simulink model "WelcomeFwdStEnCtrl"  (R2018b)
settings: Solver=FixedStepDiscrete  StartTime=0.0  StopTime=10.0  FixedStep=0.01  RelTol=1e-3
undefined symbols (not defined in the file or in its folder): data, KeSMSw4SSecRwLtStLgrstOtwdInwdClosePos1_Val, KeSMSw4SSecRwLtStLgrstUpwdDnwdClosePos1_Val, KeSMSw4SSecRwLtStLgrstUpwdDnwdClosePos2_Val, KeSMSw4SSecRwRtStLgrstOtwdInwdClosePos1_Val, KeSMSw4SSecRwRtStLgrstUpwdDnwdClosePos1_Val, KeSMSw4SSecRwRtStLgrstUpwdDnwdClosePos2_Val, SecRwLtStBkReclnEn_Clear, SecRwLtStBkReclnEn_Set, SecRwLtStFtrstEn_Clear, SecRwLtStFtrstEn_Set, SecRwLtStFwdBkwdEn_Clear, SecRwLtStFwdBkwdEn_Set, SecRwLtStHdrstFwdBkwdEn_Clear, SecRwLtStHdrstFwdBkwdEn_Set, SecRwLtStHdrstUpwdDnwdEn_Clear, SecRwLtStHdrstUpwdDnwdEn_Set, SecRwLtStLgrstInwdOtwdEn_Clear, SecRwLtStLgrstInwdOtwdEn_Set, SecRwLtStLgrstUpwdDnwdEn_Clear, SecRwLtStLgrstUpwdDnwdEn_Set, SecRwRtStBkReclnEn_Clear, SecRwRtStBkReclnEn_Set, SecRwRtStFtrstEn_Clear, SecRwRtStFtrstEn_Set, SecRwRtStFwdBkwdEn_Clear, SecRwRtStFwdBkwdEn_Set, SecRwRtStHdrstFwdBkwdEn_Clear, SecRwRtStHdrstFwdBkwdEn_Set, SecRwRtStHdrstUpwdDnwdEn_Clear, SecRwRtStHdrstUpwdDnwdEn_Set, SecRwRtStLgrstInwdOtwdEn_Clear, SecRwRtStLgrstInwdOtwdEn_Set, SecRwRtStLgrstUpwdDnwdEn_Clear, SecRwRtStLgrstUpwdDnwdEn_Set
libraries: simulink x1
settings Model: ModifiedHistory=2023.8.1 V2.0.0 CR421790 增加模式21-26  Creator=sn2xws  LastModifiedBy=sn2xws
settings DataIOCC: SaveFormat=StructureWithTime
settings OptimizationCC: DefaultParameterBehavior=Inlined  EnhancedBackFolding=on  PassReuseOutputArgsAs=Individual arguments  ZeroExternalMemoryAtStartup=off  ZeroInternalMemoryAtStartup=off  OptimizeBlockOrder=speed  DifferentSizesBufferReuse=on  OptimizationCustomize=off
settings DebuggingCC: ParameterTunabilityLossMsg=error
settings SFSimCC: MATLABDynamicMemAlloc=off
settings RTWCC: SystemTargetFile=autosar.tlc  GenCodeOnly=on  TemplateMakefile=ert_default_tmf  Description=AUTOSAR  GenerateReport=on  IncludeHyperlinkInReport=on  LaunchReport=on  GenerateTraceInfo=on  GenerateTraceReport=on  GenerateTraceReportSl=on  GenerateTraceReportSf=on  GenerateTraceReportEml=on  GenerateCodeMetricsReport=on
settings CodeAppCC: ForceParamTrailComments=on  IgnoreCustomStorageClasses=off  OperatorAnnotations=on  SimulinkDataObjDesc=on  SFDataObjDesc=on  InsertBlockDesc=on
settings STFCustomTargetCC: TargetLangStandard=C99 (ISO)  MultiwordLength=256  ParMdlRefBuildCompliant=on  CompOptLevelCompliant=on  IncludeMdlTerminateFcn=off  CombineOutputUpdateFcns=on  SuppressErrorStatus=on  ERTCustomFileBanners=on  SupportNonFinite=off  SupportComplex=off  SupportContinuousTime=off  SupportNonInlinedSFcns=off  RemoveResetFunc=on  MATLABClassNameForMDSCustomization=Simulink.SoftwareTarget.ERTCustomization  AutosarCompliant=on  UseToolchainInfoCompliant=on  LookupTableObjectStructAxisOrder=2,1,3,4,...  LUTObjectStructOrderEvenSpacing=Size,Table,Breakpoints  SystemTargetFile=autosar.tlc
settings ERTTargetCC: TargetLangStandard=C99 (ISO)  ConcurrentExecutionCompliant=off  IncludeMdlTerminateFcn=off  SuppressErrorStatus=on  SupportNonFinite=off  SupportComplex=off  ModelStepFunctionPrototypeControlCompliant=off  CPPClassGenCompliant=off  AutosarCompliant=on  LookupTableObjectStructAxisOrder=2,1,3,4,...  LUTObjectStructOrderEvenSpacing=Size,Table,Breakpoints  InlinedParameterPlacement=NonHierarchical  ERTCustomFileTemplate=example_file_process.tlc  ERTFilePackagingFormat=Compact

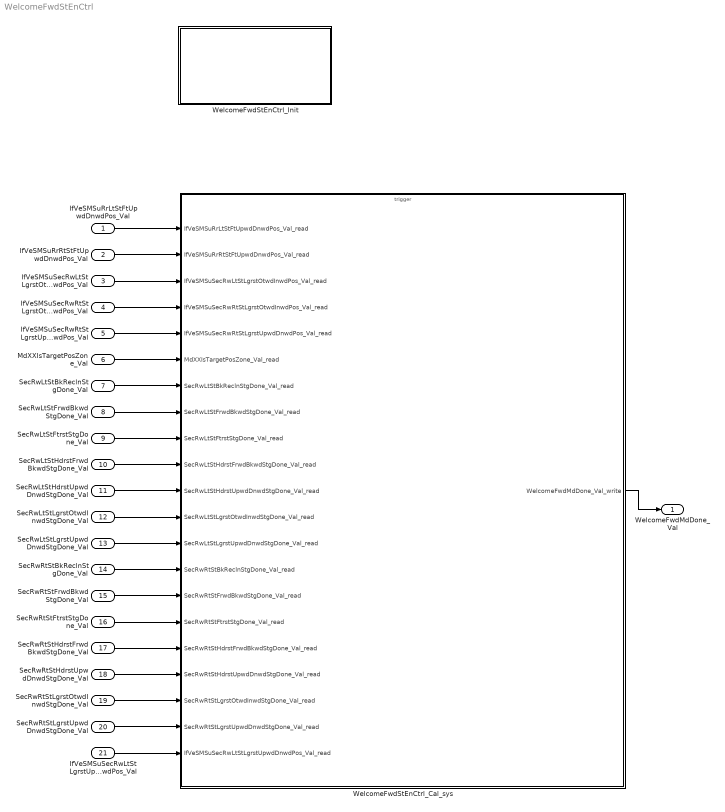
== system WelcomeFwdStEnCtrl ==
  IfVeSMSuRrLtStFtUpwdDnwdPos_Val : Inport  OutDataTypeStr=uint16  PortDimensions=1
  IfVeSMSuRrRtStFtUpwdDnwdPos_Val : Inport  Port=2  OutDataTypeStr=uint16  PortDimensions=1
  IfVeSMSuSecRwLtStLgrstOtwdInwdPos_Val : Inport  Port=3  OutDataTypeStr=uint16  PortDimensions=1
  IfVeSMSuSecRwRtStLgrstOtwdInwdPos_Val : Inport  Port=4  OutDataTypeStr=uint16  PortDimensions=1
  IfVeSMSuSecRwRtStLgrstUpwdDnwdPos_Val : Inport  Port=5  OutDataTypeStr=uint16  PortDimensions=1
  MdXXIsTargetPosZone_Val : Inport  Port=6  OutDataTypeStr=uint32  PortDimensions=1
  SecRwLtStBkReclnStgDone_Val : Inport  Port=7  OutDataTypeStr=boolean  PortDimensions=1
  SecRwLtStFrwdBkwdStgDone_Val : Inport  Port=8  OutDataTypeStr=boolean  PortDimensions=1
  SecRwLtStFtrstStgDone_Val : Inport  Port=9  OutDataTypeStr=boolean  PortDimensions=1
  SecRwLtStHdrstFrwdBkwdStgDone_Val : Inport  Port=10  OutDataTypeStr=boolean  PortDimensions=1
  SecRwLtStHdrstUpwdDnwdStgDone_Val : Inport  Port=11  OutDataTypeStr=boolean  PortDimensions=1
  SecRwLtStLgrstOtwdInwdStgDone_Val : Inport  Port=12  OutDataTypeStr=boolean  PortDimensions=1
  SecRwLtStLgrstUpwdDnwdStgDone_Val : Inport  Port=13  OutDataTypeStr=boolean  PortDimensions=1
  SecRwRtStBkReclnStgDone_Val : Inport  Port=14  OutDataTypeStr=boolean  PortDimensions=1
  SecRwRtStFrwdBkwdStgDone_Val : Inport  Port=15  OutDataTypeStr=boolean  PortDimensions=1
  SecRwRtStFtrstStgDone_Val : Inport  Port=16  OutDataTypeStr=boolean  PortDimensions=1
  SecRwRtStHdrstFrwdBkwdStgDone_Val : Inport  Port=17  OutDataTypeStr=boolean  PortDimensions=1
  SecRwRtStHdrstUpwdDnwdStgDone_Val : Inport  Port=18  OutDataTypeStr=boolean  PortDimensions=1
  SecRwRtStLgrstOtwdInwdStgDone_Val : Inport  Port=19  OutDataTypeStr=boolean  PortDimensions=1
  SecRwRtStLgrstUpwdDnwdStgDone_Val : Inport  Port=20  OutDataTypeStr=boolean  PortDimensions=1
  IfVeSMSuSecRwLtStLgrstUpwdDnwdPos_Val : Inport  Port=21  OutDataTypeStr=uint16  PortDimensions=1
  WelcomeFwdStEnCtrl_Cal_sys : Subsystem
  WelcomeFwdStEnCtrl_Init : Subsystem
  WelcomeFwdMdDone_Val : Outport  OutDataTypeStr=uint8  PortDimensions=1
  wires:
  IfVeSMSuRrLtStFtUpwdDnwdPos_Val/1 -> WelcomeFwdStEnCtrl_Cal_sys/1(IfVeSMSuRrLtStFtUpwdDnwdPos_Val_read)
  IfVeSMSuRrRtStFtUpwdDnwdPos_Val/1 -> WelcomeFwdStEnCtrl_Cal_sys/2(IfVeSMSuRrRtStFtUpwdDnwdPos_Val_read)
  IfVeSMSuSecRwLtStLgrstOtwdInwdPos_Val/1 -> WelcomeFwdStEnCtrl_Cal_sys/3(IfVeSMSuSecRwLtStLgrstOtwdInwdPos_Val_read)
  IfVeSMSuSecRwRtStLgrstOtwdInwdPos_Val/1 -> WelcomeFwdStEnCtrl_Cal_sys/4(IfVeSMSuSecRwRtStLgrstOtwdInwdPos_Val_read)
  IfVeSMSuSecRwRtStLgrstUpwdDnwdPos_Val/1 -> WelcomeFwdStEnCtrl_Cal_sys/5(IfVeSMSuSecRwRtStLgrstUpwdDnwdPos_Val_read)
  MdXXIsTargetPosZone_Val/1 -> WelcomeFwdStEnCtrl_Cal_sys/6(MdXXIsTargetPosZone_Val_read)
  SecRwLtStBkReclnStgDone_Val/1 -> WelcomeFwdStEnCtrl_Cal_sys/7(SecRwLtStBkReclnStgDone_Val_read)
  SecRwLtStFrwdBkwdStgDone_Val/1 -> WelcomeFwdStEnCtrl_Cal_sys/8(SecRwLtStFrwdBkwdStgDone_Val_read)
  SecRwLtStFtrstStgDone_Val/1 -> WelcomeFwdStEnCtrl_Cal_sys/9(SecRwLtStFtrstStgDone_Val_read)
  SecRwLtStHdrstFrwdBkwdStgDone_Val/1 -> WelcomeFwdStEnCtrl_Cal_sys/10(SecRwLtStHdrstFrwdBkwdStgDone_Val_read)
  SecRwLtStHdrstUpwdDnwdStgDone_Val/1 -> WelcomeFwdStEnCtrl_Cal_sys/11(SecRwLtStHdrstUpwdDnwdStgDone_Val_read)
  SecRwLtStLgrstOtwdInwdStgDone_Val/1 -> WelcomeFwdStEnCtrl_Cal_sys/12(SecRwLtStLgrstOtwdInwdStgDone_Val_read)
  SecRwLtStLgrstUpwdDnwdStgDone_Val/1 -> WelcomeFwdStEnCtrl_Cal_sys/13(SecRwLtStLgrstUpwdDnwdStgDone_Val_read)
  SecRwRtStBkReclnStgDone_Val/1 -> WelcomeFwdStEnCtrl_Cal_sys/14(SecRwRtStBkReclnStgDone_Val_read)
  SecRwRtStFrwdBkwdStgDone_Val/1 -> WelcomeFwdStEnCtrl_Cal_sys/15(SecRwRtStFrwdBkwdStgDone_Val_read)
  SecRwRtStFtrstStgDone_Val/1 -> WelcomeFwdStEnCtrl_Cal_sys/16(SecRwRtStFtrstStgDone_Val_read)
  SecRwRtStHdrstFrwdBkwdStgDone_Val/1 -> WelcomeFwdStEnCtrl_Cal_sys/17(SecRwRtStHdrstFrwdBkwdStgDone_Val_read)
  SecRwRtStHdrstUpwdDnwdStgDone_Val/1 -> WelcomeFwdStEnCtrl_Cal_sys/18(SecRwRtStHdrstUpwdDnwdStgDone_Val_read)
  SecRwRtStLgrstOtwdInwdStgDone_Val/1 -> WelcomeFwdStEnCtrl_Cal_sys/19(SecRwRtStLgrstOtwdInwdStgDone_Val_read)
  SecRwRtStLgrstUpwdDnwdStgDone_Val/1 -> WelcomeFwdStEnCtrl_Cal_sys/20(SecRwRtStLgrstUpwdDnwdStgDone_Val_read)
  WelcomeFwdStEnCtrl_Cal_sys/1(WelcomeFwdMdDone_Val_write) -> WelcomeFwdMdDone_Val/1
  IfVeSMSuSecRwLtStLgrstUpwdDnwdPos_Val/1 -> WelcomeFwdStEnCtrl_Cal_sys/21(IfVeSMSuSecRwLtStLgrstUpwdDnwdPos_Val_read)

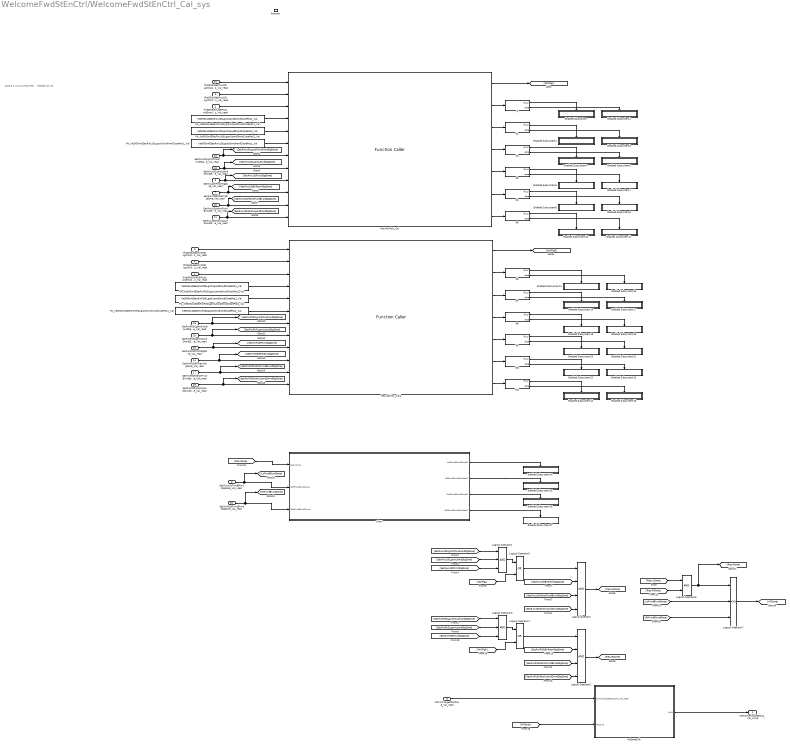
== system WelcomeFwdStEnCtrl/WelcomeFwdStEnCtrl_Cal_sys ==
  note: 2023.8.1 V2.0.0 CR421790 增加模式21-26
  IfVeSMSuRrLtStFtUpwdDnwdPos_Val_read : Inport
  IfVeSMSuRrRtStFtUpwdDnwdPos_Val_read : Inport  Port=2
  IfVeSMSuSecRwLtStLgrstOtwdInwdPos_Val_read : Inport  Port=3
  IfVeSMSuSecRwRtStLgrstOtwdInwdPos_Val_read : Inport  Port=4
  IfVeSMSuSecRwRtStLgrstUpwdDnwdPos_Val_read : Inport  Port=5
  MdXXIsTargetPosZone_Val_read : Inport  Port=6
  SecRwLtStBkReclnStgDone_Val_read : Inport  Port=7
  SecRwLtStFrwdBkwdStgDone_Val_read : Inport  Port=8
  SecRwLtStFtrstStgDone_Val_read : Inport  Port=9
  SecRwLtStHdrstFrwdBkwdStgDone_Val_read : Inport  Port=10
  SecRwLtStHdrstUpwdDnwdStgDone_Val_read : Inport  Port=11
  SecRwLtStLgrstOtwdInwdStgDone_Val_read : Inport  Port=12
  SecRwLtStLgrstUpwdDnwdStgDone_Val_read : Inport  Port=13
  SecRwRtStBkReclnStgDone_Val_read : Inport  Port=14
  SecRwRtStFrwdBkwdStgDone_Val_read : Inport  Port=15
  SecRwRtStFtrstStgDone_Val_read : Inport  Port=16
  SecRwRtStHdrstFrwdBkwdStgDone_Val_read : Inport  Port=17
  SecRwRtStHdrstUpwdDnwdStgDone_Val_read : Inport  Port=18
  SecRwRtStLgrstOtwdInwdStgDone_Val_read : Inport  Port=19
  SecRwRtStLgrstUpwdDnwdStgDone_Val_read : Inport  Port=20
  IfVeSMSuSecRwLtStLgrstUpwdDnwdPos_Val_read : Inport  Port=21
  function : TriggerPort  TriggerType=function-call  IsSimulinkFunction=on  FunctionName=WelcomeFwdStEnCtrl_Cal  VariantControl=(inherit)
  Chart : Stateflow chart  TreatAsAtomicUnit=on
  Enabled Subsystem : Subsystem  TreatAsAtomicUnit=on
  Enabled Subsystem1 : Subsystem  TreatAsAtomicUnit=on
  Enabled Subsystem10 : Subsystem  TreatAsAtomicUnit=on
  Enabled Subsystem11 : Subsystem  TreatAsAtomicUnit=on
  Enabled Subsystem12 : Subsystem  TreatAsAtomicUnit=on
  Enabled Subsystem13 : Subsystem  TreatAsAtomicUnit=on
  Enabled Subsystem14 : Subsystem  TreatAsAtomicUnit=on
  Enabled Subsystem15 : Subsystem  TreatAsAtomicUnit=on
  Enabled Subsystem16 : Subsystem  TreatAsAtomicUnit=on
  Enabled Subsystem17 : Subsystem  TreatAsAtomicUnit=on
  Enabled Subsystem18 : Subsystem  TreatAsAtomicUnit=on
  Enabled Subsystem19 : Subsystem  TreatAsAtomicUnit=on
  Enabled Subsystem2 : Subsystem  TreatAsAtomicUnit=on
  Enabled Subsystem20 : Subsystem  TreatAsAtomicUnit=on
  Enabled Subsystem21 : Subsystem  TreatAsAtomicUnit=on
  Enabled Subsystem22 : Subsystem  TreatAsAtomicUnit=on
  Enabled Subsystem23 : Subsystem  TreatAsAtomicUnit=on
  Enabled Subsystem24 : Subsystem  TreatAsAtomicUnit=on
  Enabled Subsystem25 : Subsystem  TreatAsAtomicUnit=on
  Enabled Subsystem26 : Subsystem  TreatAsAtomicUnit=on
  Enabled Subsystem27 : Subsystem  TreatAsAtomicUnit=on
  Enabled Subsystem3 : Subsystem  TreatAsAtomicUnit=on
  Enabled Subsystem4 : Subsystem  TreatAsAtomicUnit=on
  Enabled Subsystem5 : Subsystem  TreatAsAtomicUnit=on
  Enabled Subsystem6 : Subsystem  TreatAsAtomicUnit=on
  Enabled Subsystem7 : Subsystem  TreatAsAtomicUnit=on
  Enabled Subsystem8 : Subsystem  TreatAsAtomicUnit=on
  Enabled Subsystem9 : Subsystem  TreatAsAtomicUnit=on
  If{,1..11} (12 alike) : If  IfExpression=u1
  Logical Operator : Logic  Inputs=4  AllPortsSameDT=off  OutDataTypeStr=boolean
  Logical Operator1 : Logic  Inputs=3  AllPortsSameDT=off  OutDataTypeStr=boolean
  Logical Operator2 : Logic  Inputs=4  AllPortsSameDT=off  OutDataTypeStr=boolean
  Logical Operator3 : Logic  Inputs=3  AllPortsSameDT=off  OutDataTypeStr=boolean
  Logical Operator4 : Logic  Operator=OR  AllPortsSameDT=off  OutDataTypeStr=boolean
  Logical Operator5 : Logic  Operator=OR  AllPortsSameDT=off  OutDataTypeStr=boolean
  Logical Operator6 : Logic  AllPortsSameDT=off  OutDataTypeStr=boolean
  Logical Operator7 : Logic  Inputs=3  AllPortsSameDT=off  OutDataTypeStr=boolean
  MdDoneChk : Subsystem  TreatAsAtomicUnit=on
      settings: RTWSystemCode=Nonreusable function  RTWFcnNameOpts=Use subsystem name
  PA_KeSMSw4SSecRwLtStLgrstOtwdInwdClosePos1_Val : Constant  Value=KeSMSw4SSecRwLtStLgrstOtwdInwdClosePos1_Val
  PA_KeSMSw4SSecRwLtStLgrstUpwdDnwdClosePos1_Val : Constant  Value=KeSMSw4SSecRwLtStLgrstUpwdDnwdClosePos1_Val
  PA_KeSMSw4SSecRwLtStLgrstUpwdDnwdClosePos2_Val : Constant  Value=KeSMSw4SSecRwLtStLgrstUpwdDnwdClosePos2_Val
  PA_KeSMSw4SSecRwRtStLgrstOtwdInwdClosePos1_Val : Constant  Value=KeSMSw4SSecRwRtStLgrstOtwdInwdClosePos1_Val
  PA_KeSMSw4SSecRwRtStLgrstUpwdDnwdClosePos1_Val : Constant  Value=KeSMSw4SSecRwRtStLgrstUpwdDnwdClosePos1_Val
  PA_KeSMSw4SSecRwRtStLgrstUpwdDnwdClosePos2_Val : Constant  Value=KeSMSw4SSecRwRtStLgrstUpwdDnwdClosePos2_Val
  Recv4sFlow_Cal : FunctionCaller  FunctionPrototype=[Failflg,LgrstInwdOtwdEn,LgrstUpwdDnwdEn,FtrstEn,BkReclnEn,HdrstFrwdBkwdEn,HdrstUpwdDnwdEn] = Recv4sFlow_Cal(LgrstUpwdDnwdPos,LgrstOtwdInwdPos,FtUpwdDnwdPos,CloseDnwdPos1,CloseDnwdPos2,CloseOtwdPos1,LgrstInwdStgDone,LgrstUpwdStgDone,FtrstStgDone,BkReclnStgDone,HdrstFwdBkwdStgDone,HdrstupwdDnwdStgDone)  InputArgumentSpecifications=uint16(1), uint16(1), uint16(1), uint16(1), uint16(1), uint16(1), boolean(true), boolean(true), boolean(true), boolean(true), boolean(true), boolean(true)  OutputArgumentSpecifications=boolean(true), boolean(true), boolean(true), boolean(true), boolean(true), boolean(true), boolean(true)
  Recv4sFlow_Cal1 : FunctionCaller  FunctionPrototype=[Failflg,LgrstInwdOtwdEn,LgrstUpwdDnwdEn,FtrstEn,BkReclnEn,HdrstFrwdBkwdEn,HdrstUpwdDnwdEn] = Recv4sFlow_Cal(LgrstUpwdDnwdPos,LgrstOtwdInwdPos,FtUpwdDnwdPos,CloseDnwdPos1,CloseDnwdPos2,CloseOtwdPos1,LgrstInwdStgDone,LgrstUpwdStgDone,FtrstStgDone,BkReclnStgDone,HdrstFwdBkwdStgDone,HdrstupwdDnwdStgDone)  InputArgumentSpecifications=uint16(1), uint16(1), uint16(1), uint16(1), uint16(1), uint16(1), boolean(true), boolean(true), boolean(true), boolean(true), boolean(true), boolean(true)  OutputArgumentSpecifications=boolean(true), boolean(true), boolean(true), boolean(true), boolean(true), boolean(true), boolean(true)
  WelcomeFwdMdDone_Val_write : Outport
      settings: EnsureOutportIsVirtual=on
  wires:
  IfVeSMSuSecRwRtStLgrstOtwdInwdPos_Val_read/1 -> Recv4sFlow_Cal1/2
  IfVeSMSuSecRwRtStLgrstUpwdDnwdPos_Val_read/1 -> Recv4sFlow_Cal1/1
  SecRwLtStFrwdBkwdStgDone_Val_read/1 -> [LtFrwdBkwdDone], Chart/2(LtStFrwdBkwdDone)
  SecRwRtStFrwdBkwdStgDone_Val_read/1 -> [RtFrwdBkwdDone], Chart/3(RtStFrwdBkwdDone)
  IfVeSMSuSecRwLtStLgrstOtwdInwdPos_Val_read/1 -> Recv4sFlow_Cal/2
  IfVeSMSuRrLtStFtUpwdDnwdPos_Val_read/1 -> Recv4sFlow_Cal/3
  IfVeSMSuRrRtStFtUpwdDnwdPos_Val_read/1 -> Recv4sFlow_Cal1/3
  SecRwLtStLgrstOtwdInwdStgDone_Val_read/1 -> [SecRwLtStLgrstOtwdInwdStgDone], Recv4sFlow_Cal/7
  SecRwLtStLgrstUpwdDnwdStgDone_Val_read/1 -> [SecRwLtStLgrstUpwdStgDone], Recv4sFlow_Cal/8
  SecRwLtStFtrstStgDone_Val_read/1 -> [SecRwLtStFtrstStgDone], Recv4sFlow_Cal/9
  SecRwLtStBkReclnStgDone_Val_read/1 -> [SecRwLtStBkReclnStgDone], Recv4sFlow_Cal/10
  SecRwLtStHdrstFrwdBkwdStgDone_Val_read/1 -> [SecRwLtStHdrstFrwdBkwdStgDone], Recv4sFlow_Cal/11
  SecRwLtStHdrstUpwdDnwdStgDone_Val_read/1 -> [SecRwLtStHdrstUpwdDnwdStgDone], Recv4sFlow_Cal/12
  SecRwRtStLgrstOtwdInwdStgDone_Val_read/1 -> [SecRwRtStLgrstOtwdInwdStgDone], Recv4sFlow_Cal1/7
  SecRwRtStLgrstUpwdDnwdStgDone_Val_read/1 -> [SecRwRtStLgrstUpwdStgDone], Recv4sFlow_Cal1/8
  SecRwRtStFtrstStgDone_Val_read/1 -> [SecRwRtStFtrstStgDone], Recv4sFlow_Cal1/9
  SecRwRtStBkReclnStgDone_Val_read/1 -> [SecRwRtStBkReclnStgDone], Recv4sFlow_Cal1/10
  SecRwRtStHdrstFrwdBkwdStgDone_Val_read/1 -> [SecRwRtStHdrstFrwdBkwdStgDone], Recv4sFlow_Cal1/11
  SecRwRtStHdrstUpwdDnwdStgDone_Val_read/1 -> [SecRwRtStHdrstUpwdDnwdStgDone], Recv4sFlow_Cal1/12
  Recv4sFlow_Cal/1 -> [FailFlgL]
  Recv4sFlow_Cal1/1 -> [FailFlgR]
  [SecRwLtStHdrstFrwdBkwdStgDone] -> Logical Operator/3
  [SecRwLtStLgrstUpwdStgDone] -> Logical Operator1/2
  Logical Operator1/1 -> Logical Operator5/1
  [FailFlgL] -> Logical Operator5/2
  Logical Operator5/1 -> Logical Operator/1
  [SecRwLtStHdrstUpwdDnwdStgDone] -> Logical Operator/4
  [SecRwLtStLgrstOtwdInwdStgDone] -> Logical Operator1/1
  Logical Operator/1 -> [RecvLDone]
  [SecRwLtStBkReclnStgDone] -> Logical Operator/2
  [SecRwLtStFtrstStgDone] -> Logical Operator1/3
  Recv4sFlow_Cal/2 -> If/1
  Recv4sFlow_Cal/3 -> If1/1
  Recv4sFlow_Cal/4 -> If2/1
  Recv4sFlow_Cal/5 -> If3/1
  Recv4sFlow_Cal/6 -> If4/1
  Recv4sFlow_Cal/7 -> If5/1
  Recv4sFlow_Cal1/2 -> If6/1
  Recv4sFlow_Cal1/3 -> If7/1
  Recv4sFlow_Cal1/4 -> If8/1
  Recv4sFlow_Cal1/5 -> If9/1
  Recv4sFlow_Cal1/6 -> If10/1
  Recv4sFlow_Cal1/7 -> If11/1
  If/1 -> Enabled Subsystem/Action
  If/2 -> Enabled Subsystem1/Action
  If1/1 -> Enabled Subsystem2/Action
  If1/2 -> Enabled Subsystem3/Action
  If2/1 -> Enabled Subsystem4/Action
  If2/2 -> Enabled Subsystem5/Action
  If3/1 -> Enabled Subsystem6/Action
  If3/2 -> Enabled Subsystem7/Action
  If4/1 -> Enabled Subsystem8/Action
  If4/2 -> Enabled Subsystem9/Action
  If5/1 -> Enabled Subsystem10/Action
  If5/2 -> Enabled Subsystem11/Action
  If6/1 -> Enabled Subsystem12/Action
  If6/2 -> Enabled Subsystem13/Action
  If7/1 -> Enabled Subsystem16/Action
  If7/2 -> Enabled Subsystem17/Action
  If8/1 -> Enabled Subsystem18/Action
  If8/2 -> Enabled Subsystem19/Action
  If9/1 -> Enabled Subsystem20/Action
  If9/2 -> Enabled Subsystem21/Action
  If10/1 -> Enabled Subsystem22/Action
  If10/2 -> Enabled Subsystem23/Action
  If11/1 -> Enabled Subsystem14/Action
  If11/2 -> Enabled Subsystem15/Action
  [SecRwRtStFtrstStgDone] -> Logical Operator3/3
  [SecRwRtStBkReclnStgDone] -> Logical Operator2/2
  Logical Operator2/1 -> [RecvRDone]
  [SecRwRtStLgrstOtwdInwdStgDone] -> Logical Operator3/1
  [SecRwRtStHdrstUpwdDnwdStgDone] -> Logical Operator2/4
  Logical Operator4/1 -> Logical Operator2/1
  [FailFlgR] -> Logical Operator4/2
  Logical Operator3/1 -> Logical Operator4/1
  [SecRwRtStLgrstUpwdStgDone] -> Logical Operator3/2
  [SecRwRtStHdrstFrwdBkwdStgDone] -> Logical Operator2/3
  [RecvLDone] -> Logical Operator6/1
  [RecvRDone] -> Logical Operator6/2
  Logical Operator6/1 -> [RecvDone], Logical Operator7/1
  Logical Operator7/1 -> [AllDone]
  [RecvDone] -> Chart/1(RecvDone)
  [LtFrwdBkwdDone] -> Logical Operator7/2
  [RtFrwdBkwdDone] -> Logical Operator7/3
  IfVeSMSuSecRwLtStLgrstUpwdDnwdPos_Val_read/1 -> Recv4sFlow_Cal/1
  PA_KeSMSw4SSecRwLtStLgrstUpwdDnwdClosePos1_Val/1 -> Recv4sFlow_Cal/4
  PA_KeSMSw4SSecRwLtStLgrstUpwdDnwdClosePos2_Val/1 -> Recv4sFlow_Cal/5
  PA_KeSMSw4SSecRwLtStLgrstOtwdInwdClosePos1_Val/1 -> Recv4sFlow_Cal/6
  PA_KeSMSw4SSecRwRtStLgrstUpwdDnwdClosePos1_Val/1 -> Recv4sFlow_Cal1/4
  PA_KeSMSw4SSecRwRtStLgrstUpwdDnwdClosePos2_Val/1 -> Recv4sFlow_Cal1/5
  PA_KeSMSw4SSecRwRtStLgrstOtwdInwdClosePos1_Val/1 -> Recv4sFlow_Cal1/6
  MdXXIsTargetPosZone_Val_read/1 -> MdDoneChk/1(MdXXIsTargetPosZone_Val_read)
  MdDoneChk/1(Out1) -> WelcomeFwdMdDone_Val_write/1
  [AllDone] -> MdDoneChk/2(AllDone)
  Chart/1(LtStFrwdBkwdEnSet()) -> Enabled Subsystem24/Trigger
  Chart/2(LtStFrwdBkwdEnClear()) -> Enabled Subsystem25/Trigger
  Chart/3(RtStFrwdBkwdEnSet()) -> Enabled Subsystem26/Trigger
  Chart/4(RtStFrwdBkwdEnClear()) -> Enabled Subsystem27/Trigger

== system WelcomeFwdStEnCtrl/WelcomeFwdStEnCtrl_Init ==
  Event Listener : EventListener  EventName=reset

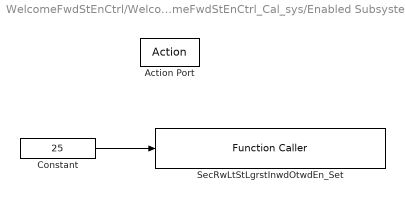
== system WelcomeFwdStEnCtrl/WelcomeFwdStEnCtrl_Cal_sys/Enabled Subsystem ==
  Action Port : ActionPort  ActionType=then
  Constant : Constant  Value=25  OutDataTypeStr=uint8
  SecRwLtStLgrstInwdOtwdEn_Set : FunctionCaller  FunctionPrototype=SecRwLtStLgrstInwdOtwdEn_Set(data)  InputArgumentSpecifications=uint8(1)
  wires:
  Constant/1 -> SecRwLtStLgrstInwdOtwdEn_Set/1

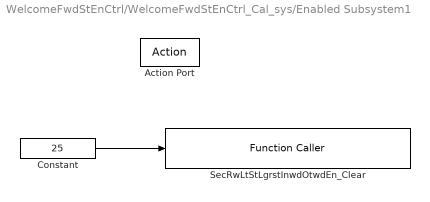
== system WelcomeFwdStEnCtrl/WelcomeFwdStEnCtrl_Cal_sys/Enabled Subsystem1 ==
  Action Port : ActionPort  ActionType=else
  Constant : Constant  Value=25  OutDataTypeStr=uint8
  SecRwLtStLgrstInwdOtwdEn_Clear : FunctionCaller  FunctionPrototype=SecRwLtStLgrstInwdOtwdEn_Clear(data)  InputArgumentSpecifications=uint8(1)
  wires:
  Constant/1 -> SecRwLtStLgrstInwdOtwdEn_Clear/1

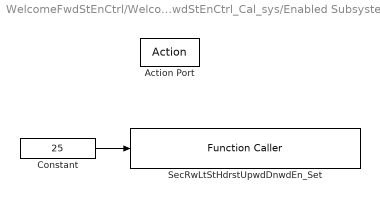
== system WelcomeFwdStEnCtrl/WelcomeFwdStEnCtrl_Cal_sys/Enabled Subsystem10 ==
  Action Port : ActionPort  ActionType=then
  Constant : Constant  Value=25  OutDataTypeStr=uint8
  SecRwLtStHdrstUpwdDnwdEn_Set : FunctionCaller  FunctionPrototype=SecRwLtStHdrstUpwdDnwdEn_Set(data)  InputArgumentSpecifications=uint8(1)
  wires:
  Constant/1 -> SecRwLtStHdrstUpwdDnwdEn_Set/1

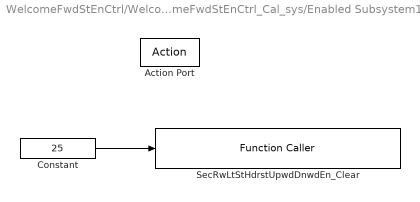
== system WelcomeFwdStEnCtrl/WelcomeFwdStEnCtrl_Cal_sys/Enabled Subsystem11 ==
  Action Port : ActionPort  ActionType=else
  Constant : Constant  Value=25  OutDataTypeStr=uint8
  SecRwLtStHdrstUpwdDnwdEn_Clear : FunctionCaller  FunctionPrototype=SecRwLtStHdrstUpwdDnwdEn_Clear(data)  InputArgumentSpecifications=uint8(1)
  wires:
  Constant/1 -> SecRwLtStHdrstUpwdDnwdEn_Clear/1

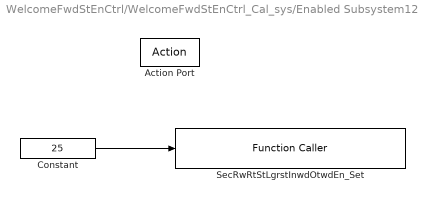
== system WelcomeFwdStEnCtrl/WelcomeFwdStEnCtrl_Cal_sys/Enabled Subsystem12 ==
  Action Port : ActionPort  ActionType=then
  Constant : Constant  Value=25  OutDataTypeStr=uint8
  SecRwRtStLgrstInwdOtwdEn_Set : FunctionCaller  FunctionPrototype=SecRwRtStLgrstInwdOtwdEn_Set(data)  InputArgumentSpecifications=uint8(1)
  wires:
  Constant/1 -> SecRwRtStLgrstInwdOtwdEn_Set/1

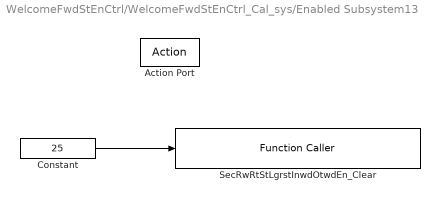
== system WelcomeFwdStEnCtrl/WelcomeFwdStEnCtrl_Cal_sys/Enabled Subsystem13 ==
  Action Port : ActionPort  ActionType=else
  Constant : Constant  Value=25  OutDataTypeStr=uint8
  SecRwRtStLgrstInwdOtwdEn_Clear : FunctionCaller  FunctionPrototype=SecRwRtStLgrstInwdOtwdEn_Clear(data)  InputArgumentSpecifications=uint8(1)
  wires:
  Constant/1 -> SecRwRtStLgrstInwdOtwdEn_Clear/1

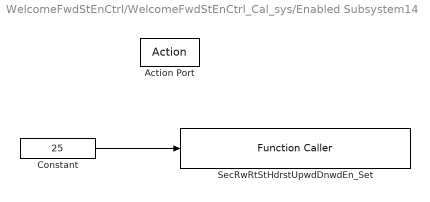
== system WelcomeFwdStEnCtrl/WelcomeFwdStEnCtrl_Cal_sys/Enabled Subsystem14 ==
  Action Port : ActionPort  ActionType=then
  Constant : Constant  Value=25  OutDataTypeStr=uint8
  SecRwRtStHdrstUpwdDnwdEn_Set : FunctionCaller  FunctionPrototype=SecRwRtStHdrstUpwdDnwdEn_Set(data)  InputArgumentSpecifications=uint8(1)
  wires:
  Constant/1 -> SecRwRtStHdrstUpwdDnwdEn_Set/1

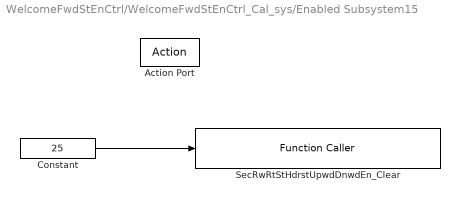
== system WelcomeFwdStEnCtrl/WelcomeFwdStEnCtrl_Cal_sys/Enabled Subsystem15 ==
  Action Port : ActionPort  ActionType=else
  Constant : Constant  Value=25  OutDataTypeStr=uint8
  SecRwRtStHdrstUpwdDnwdEn_Clear : FunctionCaller  FunctionPrototype=SecRwRtStHdrstUpwdDnwdEn_Clear(data)  InputArgumentSpecifications=uint8(1)
  wires:
  Constant/1 -> SecRwRtStHdrstUpwdDnwdEn_Clear/1

== system WelcomeFwdStEnCtrl/WelcomeFwdStEnCtrl_Cal_sys/Enabled Subsystem16 ==
  Action Port : ActionPort  ActionType=then
  Constant : Constant  Value=25  OutDataTypeStr=uint8
  SecRwRtStLgrstUpwdDnwdEn_Set : FunctionCaller  FunctionPrototype=SecRwRtStLgrstUpwdDnwdEn_Set(data)  InputArgumentSpecifications=uint8(1)
  wires:
  Constant/1 -> SecRwRtStLgrstUpwdDnwdEn_Set/1

== system WelcomeFwdStEnCtrl/WelcomeFwdStEnCtrl_Cal_sys/Enabled Subsystem17 ==
  Action Port : ActionPort  ActionType=else
  Constant : Constant  Value=25  OutDataTypeStr=uint8
  SecRwRtStLgrstUpwdDnwdEn_Clear : FunctionCaller  FunctionPrototype=SecRwRtStLgrstUpwdDnwdEn_Clear(data)  InputArgumentSpecifications=uint8(1)
  wires:
  Constant/1 -> SecRwRtStLgrstUpwdDnwdEn_Clear/1

== system WelcomeFwdStEnCtrl/WelcomeFwdStEnCtrl_Cal_sys/Enabled Subsystem18 ==
  Action Port : ActionPort  ActionType=then
  Constant : Constant  Value=25  OutDataTypeStr=uint8
  SecRwRtStFtrstEn_Set : FunctionCaller  FunctionPrototype=SecRwRtStFtrstEn_Set(data)  InputArgumentSpecifications=uint8(1)
  wires:
  Constant/1 -> SecRwRtStFtrstEn_Set/1

== system WelcomeFwdStEnCtrl/WelcomeFwdStEnCtrl_Cal_sys/Enabled Subsystem19 ==
  Action Port : ActionPort  ActionType=else
  Constant : Constant  Value=25  OutDataTypeStr=uint8
  SecRwRtStFtrstEn_Clear : FunctionCaller  FunctionPrototype=SecRwRtStFtrstEn_Clear(data)  InputArgumentSpecifications=uint8(1)
  wires:
  Constant/1 -> SecRwRtStFtrstEn_Clear/1

== system WelcomeFwdStEnCtrl/WelcomeFwdStEnCtrl_Cal_sys/Enabled Subsystem2 ==
  Action Port : ActionPort  ActionType=then
  Constant : Constant  Value=25  OutDataTypeStr=uint8
  SecRwLtStLgrstUpwdDnwdEn_Set : FunctionCaller  FunctionPrototype=SecRwLtStLgrstUpwdDnwdEn_Set(data)  InputArgumentSpecifications=uint8(1)
  wires:
  Constant/1 -> SecRwLtStLgrstUpwdDnwdEn_Set/1

== system WelcomeFwdStEnCtrl/WelcomeFwdStEnCtrl_Cal_sys/Enabled Subsystem20 ==
  Action Port : ActionPort  ActionType=then
  Constant : Constant  Value=25  OutDataTypeStr=uint8
  SecRwRtStBkReclnEn_Set : FunctionCaller  FunctionPrototype=SecRwRtStBkReclnEn_Set(data)  InputArgumentSpecifications=uint8(1)
  wires:
  Constant/1 -> SecRwRtStBkReclnEn_Set/1

== system WelcomeFwdStEnCtrl/WelcomeFwdStEnCtrl_Cal_sys/Enabled Subsystem21 ==
  Action Port : ActionPort  ActionType=else
  Constant : Constant  Value=25  OutDataTypeStr=uint8
  SecRwRtStBkReclnEn_Clear : FunctionCaller  FunctionPrototype=SecRwRtStBkReclnEn_Clear(data)  InputArgumentSpecifications=uint8(1)
  wires:
  Constant/1 -> SecRwRtStBkReclnEn_Clear/1

== system WelcomeFwdStEnCtrl/WelcomeFwdStEnCtrl_Cal_sys/Enabled Subsystem22 ==
  Action Port : ActionPort  ActionType=then
  Constant : Constant  Value=25  OutDataTypeStr=uint8
  SecRwRtStHdrstFwdBkwdEn_Set : FunctionCaller  FunctionPrototype=SecRwRtStHdrstFwdBkwdEn_Set(data)  InputArgumentSpecifications=uint8(1)
  wires:
  Constant/1 -> SecRwRtStHdrstFwdBkwdEn_Set/1

== system WelcomeFwdStEnCtrl/WelcomeFwdStEnCtrl_Cal_sys/Enabled Subsystem23 ==
  Action Port : ActionPort  ActionType=else
  Constant : Constant  Value=25  OutDataTypeStr=uint8
  SecRwRtStHdrstFwdBkwdEn_Clear : FunctionCaller  FunctionPrototype=SecRwRtStHdrstFwdBkwdEn_Clear(data)  InputArgumentSpecifications=uint8(1)
  wires:
  Constant/1 -> SecRwRtStHdrstFwdBkwdEn_Clear/1

== system WelcomeFwdStEnCtrl/WelcomeFwdStEnCtrl_Cal_sys/Enabled Subsystem24 ==
  Trigger : TriggerPort  TriggerType=function-call  VariantControl=Variant  PortDimensions=1
  Constant : Constant  Value=25  OutDataTypeStr=uint8
  SecRwLtStFwdBkwdEn_Set : FunctionCaller  FunctionPrototype=SecRwLtStFwdBkwdEn_Set(data)  InputArgumentSpecifications=uint8(1)
  wires:
  Constant/1 -> SecRwLtStFwdBkwdEn_Set/1

== system WelcomeFwdStEnCtrl/WelcomeFwdStEnCtrl_Cal_sys/Enabled Subsystem25 ==
  Trigger : TriggerPort  TriggerType=function-call  VariantControl=Variant  PortDimensions=1
  Constant : Constant  Value=25  OutDataTypeStr=uint8
  SecRwLtStFwdBkwdEn_Clear : FunctionCaller  FunctionPrototype=SecRwLtStFwdBkwdEn_Clear(data)  InputArgumentSpecifications=uint8(1)
  wires:
  Constant/1 -> SecRwLtStFwdBkwdEn_Clear/1

== system WelcomeFwdStEnCtrl/WelcomeFwdStEnCtrl_Cal_sys/Enabled Subsystem26 ==
  Trigger : TriggerPort  TriggerType=function-call  VariantControl=Variant  PortDimensions=1
  Constant : Constant  Value=25  OutDataTypeStr=uint8
  SecRwRtStFwdBkwdEn_Set : FunctionCaller  FunctionPrototype=SecRwRtStFwdBkwdEn_Set(data)  InputArgumentSpecifications=uint8(1)
  wires:
  Constant/1 -> SecRwRtStFwdBkwdEn_Set/1

== system WelcomeFwdStEnCtrl/WelcomeFwdStEnCtrl_Cal_sys/Enabled Subsystem27 ==
  Trigger : TriggerPort  TriggerType=function-call  VariantControl=Variant  PortDimensions=1
  Constant : Constant  Value=25  OutDataTypeStr=uint8
  SecRwRtStFwdBkwdEn_Clear : FunctionCaller  FunctionPrototype=SecRwRtStFwdBkwdEn_Clear(data)  InputArgumentSpecifications=uint8(1)
  wires:
  Constant/1 -> SecRwRtStFwdBkwdEn_Clear/1

== system WelcomeFwdStEnCtrl/WelcomeFwdStEnCtrl_Cal_sys/Enabled Subsystem3 ==
  Action Port : ActionPort  ActionType=else
  Constant : Constant  Value=25  OutDataTypeStr=uint8
  SecRwLtStLgrstUpwdDnwdEn_Clear : FunctionCaller  FunctionPrototype=SecRwLtStLgrstUpwdDnwdEn_Clear(data)  InputArgumentSpecifications=uint8(1)
  wires:
  Constant/1 -> SecRwLtStLgrstUpwdDnwdEn_Clear/1

== system WelcomeFwdStEnCtrl/WelcomeFwdStEnCtrl_Cal_sys/Enabled Subsystem4 ==
  Action Port : ActionPort  ActionType=then
  Constant : Constant  Value=25  OutDataTypeStr=uint8
  SecRwLtStFtrstEn_Set : FunctionCaller  FunctionPrototype=SecRwLtStFtrstEn_Set(data)  InputArgumentSpecifications=uint8(1)
  wires:
  Constant/1 -> SecRwLtStFtrstEn_Set/1

== system WelcomeFwdStEnCtrl/WelcomeFwdStEnCtrl_Cal_sys/Enabled Subsystem5 ==
  Action Port : ActionPort  ActionType=else
  Constant : Constant  Value=25  OutDataTypeStr=uint8
  SecRwLtStFtrstEn_Clear : FunctionCaller  FunctionPrototype=SecRwLtStFtrstEn_Clear(data)  InputArgumentSpecifications=uint8(1)
  wires:
  Constant/1 -> SecRwLtStFtrstEn_Clear/1

== system WelcomeFwdStEnCtrl/WelcomeFwdStEnCtrl_Cal_sys/Enabled Subsystem6 ==
  Action Port : ActionPort  ActionType=then
  Constant : Constant  Value=25  OutDataTypeStr=uint8
  SecRwLtStBkReclnEn_Set : FunctionCaller  FunctionPrototype=SecRwLtStBkReclnEn_Set(data)  InputArgumentSpecifications=uint8(1)
  wires:
  Constant/1 -> SecRwLtStBkReclnEn_Set/1

== system WelcomeFwdStEnCtrl/WelcomeFwdStEnCtrl_Cal_sys/Enabled Subsystem7 ==
  Action Port : ActionPort  ActionType=else
  Constant : Constant  Value=25  OutDataTypeStr=uint8
  SecRwLtStBkReclnEn_Clear : FunctionCaller  FunctionPrototype=SecRwLtStBkReclnEn_Clear(data)  InputArgumentSpecifications=uint8(1)
  wires:
  Constant/1 -> SecRwLtStBkReclnEn_Clear/1

== system WelcomeFwdStEnCtrl/WelcomeFwdStEnCtrl_Cal_sys/Enabled Subsystem8 ==
  Action Port : ActionPort  ActionType=then
  Constant : Constant  Value=25  OutDataTypeStr=uint8
  SecRwLtStHdrstFwdBkwdEn_Set : FunctionCaller  FunctionPrototype=SecRwLtStHdrstFwdBkwdEn_Set(data)  InputArgumentSpecifications=uint8(1)
  wires:
  Constant/1 -> SecRwLtStHdrstFwdBkwdEn_Set/1

== system WelcomeFwdStEnCtrl/WelcomeFwdStEnCtrl_Cal_sys/Enabled Subsystem9 ==
  Action Port : ActionPort  ActionType=else
  Constant : Constant  Value=25  OutDataTypeStr=uint8
  SecRwLtStHdrstFwdBkwdEn_Clear : FunctionCaller  FunctionPrototype=SecRwLtStHdrstFwdBkwdEn_Clear(data)  InputArgumentSpecifications=uint8(1)
  wires:
  Constant/1 -> SecRwLtStHdrstFwdBkwdEn_Clear/1

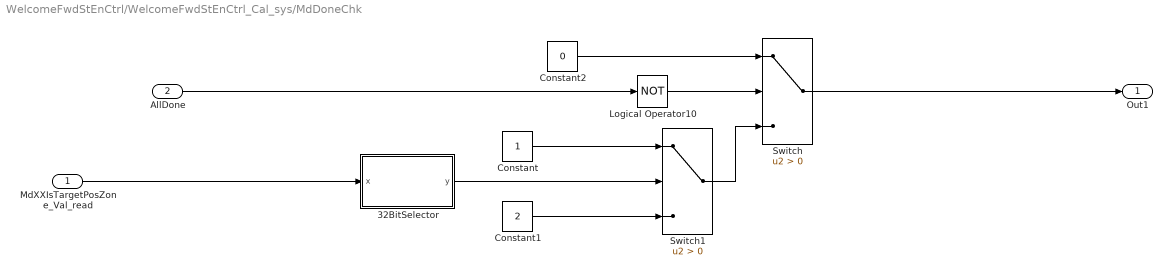
== system WelcomeFwdStEnCtrl/WelcomeFwdStEnCtrl_Cal_sys/MdDoneChk ==
  MdXXIsTargetPosZone_Val_read : Inport
  AllDone : Inport  Port=2
  32BitSelector : Subsystem  mask(32 Bit Selector){BitNum=25}
      mask prompts: BitNum "Select Bit Number"
      mask help: Allows selection of a particular bit (0-31) out of a packed word up to 32 bits long. Output will be true if the bit number selected via the mask parameter is equal to one.
      mask TypeOptions BitNum: 0 | 1 | 2 | 3 | 4 | 5 | 6 | 7 | 8 | 9 | 10 | 11 | 12 | 13 | 14 | 15 | 16 | 17 | 18 | 19 | 20 | 21 | 22 | 23 | 24 | 25 | 26 | 27 | 28 | 29 | 30 | 31
      mask Display:
      | text(0.5, 0.8,'BIT','horizontalAlignment','center')
      | text(0.5, 0.5,'SELECTOR','horizontalAlignment','center')
      | text(0.5, 0.2,['-- Bit ',char(get_param(gcb,'BitNum')),' --'],'horizontalAlignment','center')
  Constant : Constant  OutDataTypeStr=uint8
  Constant1 : Constant  Value=2  OutDataTypeStr=uint8
  Constant2 : Constant  Value=0  OutDataTypeStr=uint8
  Logical Operator10 : Logic  Operator=NOT  AllPortsSameDT=off  OutDataTypeStr=boolean
  Switch : Switch  Criteria=u2 > Threshold
  Switch1 : Switch  Criteria=u2 > Threshold
  Out1 : Outport
  wires:
  Switch1/1 -> Switch/3
  AllDone/1 -> Logical Operator10/1
  Switch/1 -> Out1/1
  MdXXIsTargetPosZone_Val_read/1 -> 32BitSelector/1(x)
  Constant2/1 -> Switch/1
  Constant1/1 -> Switch1/3
  Constant/1 -> Switch1/1
  Logical Operator10/1 -> Switch/2
  32BitSelector/1(y) -> Switch1/2

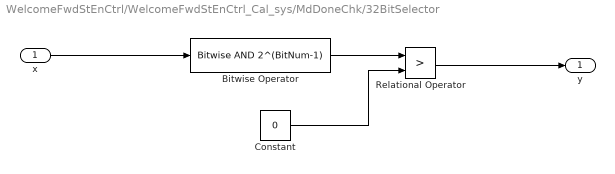
== system WelcomeFwdStEnCtrl/WelcomeFwdStEnCtrl_Cal_sys/MdDoneChk/32BitSelector ==
  x : Inport
  Bitwise Operator : simulink/Logic and Bit Operations/Bitwise Operator  logicop=AND  UseBitMask=on  BitMask=2^(BitNum-1)  BitMaskRealWorld=Stored Integer
  Constant : Constant  Value=0  OutDataTypeStr=uint32
  Relational Operator : RelationalOperator  Operator=>  OutDataTypeStr=boolean  RndMeth=Simplest
  y : Outport
  wires:
  Relational Operator/1 -> y/1
  Constant/1 -> Relational Operator/2
  x/1 -> Bitwise Operator/1
  Bitwise Operator/1 -> Relational Operator/1

== stateflow chart WelcomeFwdStEnCtrl/WelcomeFwdStEnCtrl_Cal_sys/Chart ==
  (default) -> (junction 1)
  (junction 1) -> (junction 3)
  (junction 3) -> (junction 5) [order 1] : [RecvDone &&!LtStFrwdBkwdDone]
  (junction 3) -> (junction 9) [order 2] : {LtStFrwdBkwdEnClear}
  (junction 5) -> (junction 7) : {LtStFrwdBkwdEnSet;}
  (junction 7) -> (junction 9)
  (junction 9) -> (junction 17)
  (junction 17) -> (junction 19) [order 1] : [RecvDone &&!RtStFrwdBkwdDone]
  (junction 17) -> (junction 23) [order 2] : {RtStFrwdBkwdEnClear;}
  (junction 19) -> (junction 21) : {RtStFrwdBkwdEnSet;}
  (junction 21) -> (junction 23)
  (junction 23) -> (junction 26)
  data: RecvDone input; LtStFrwdBkwdDone input; RtStFrwdBkwdDone input
  events: LtStFrwdBkwdEnSet output FUNCTION_CALL_EVENT; LtStFrwdBkwdEnClear output FUNCTION_CALL_EVENT; RtStFrwdBkwdEnSet output FUNCTION_CALL_EVENT; RtStFrwdBkwdEnClear output FUNCTION_CALL_EVENT
